simulink model "Estimador_DB_Caso_2"  (R2023a)
settings: Solver=VariableStepAuto  StartTime=0.0  StopTime=6  MaxStep=0.001  MinStep=0.0001  RelTol=1e-3  EnableMultiTasking=on
values from neighbouring files (symbols this model uses):
  A = [-1/(C1*R1) 1/(R1*C1);1/(C2*R1) -1/C2*(1/R1+1/R2)]    [MIMO_Real_Tanques.m]
  B = [1/C1 0;0 1/C2]    [MIMO_Real_Tanques.m]
  C = [1 0;0 1;0 1/R2]    [MIMO_Real_Tanques.m]
  D = [0 0;0 0;0 0]    [MIMO_Real_Tanques.m]
  K = place(A,B,PLC)    [MIMO_Real_Tanques.m]
  K0 = pinv(dcgain(ss(An,B,C,D)))*Y_inf*pinv(Q_inf)    [MIMO_Real_Tanques.m]
  Ke = place(A',C',PEE)'    [MIMO_Real_Tanques.m]
  Q1 = 3    [MIMO_Real_Tanques.m]
  Q2 = 1    [MIMO_Real_Tanques.m]
settings Model: Creator=54115  LastModifiedBy=franc
settings SolverCC: AlgebraicLoopSolver=TrustRegion
settings DataIOCC: ReturnWorkspaceOutputs=off
settings OptimizationCC: LifeSpan=inf
settings DebuggingCC: UnconnectedInputMsg=warning  UnconnectedOutputMsg=warning  UnconnectedLineMsg=warning  SFUnexpectedBacktrackingDiag=warning  SFNoUnconditionalDefaultTransitionDiag=warning  ArithmeticOperatorsInVariantConditions=warning
settings ModelReferenceCC: EnableRefExpFcnMdlSchedulingChecks=on
settings SFSimCC: SimUseLocalCustomCode=off  CustomCodeUndefinedFunction=UseInterfaceOnly
settings RTWCC: RTWUseLocalCustomCode=off
settings CodeAppCC: StateflowObjectComments=on
settings GRTTargetCC: TargetLangStandard=C89/C90 (ANSI)
settings ConfigComp: CovMetricSettings=dw  CovSaveCumulativeToWorkspaceVar=on  CovSaveSingleToWorkspaceVar=on  CovExternalEMLEnable=off

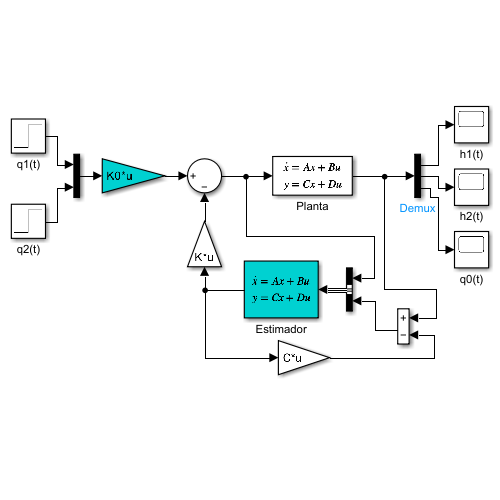
[thumbnail: Simulink's stored preview of the top-level diagram]
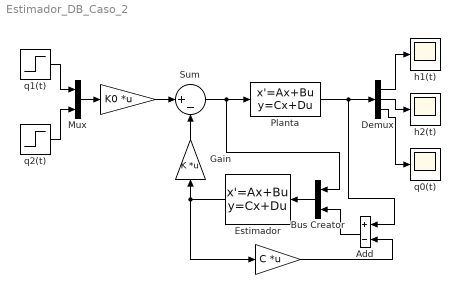
== system Estimador_DB_Caso_2 ==
  " " : Gain  Gain=K0  Multiplication=Matrix(K*u)
  "  " : Gain  Gain=C  Multiplication=Matrix(K*u)
  Add : Sum  Inputs=+-
  Bus Creator : BusCreator  Inputs=2
  Demux : Demux  Outputs=3
  Estimador : StateSpace  A=A  B=[B Ke]  C=eye(2)  D=[0 0 0 0 0;0 0 0 0 0]  InitialCondition=0
  Gain : Gain  Gain=K  Multiplication=Matrix(K*u)
  Mux : Mux  Inputs=2
  Planta : StateSpace  A=A  B=B  C=C  D=D  InitialCondition=0
  Sum : Sum  Inputs=|+-
  h1(t) : Scope
  h2(t) : Scope
  q0(t) : Scope
  q1(t) : Step  Time=0  After=Q1  SampleTime=0
  q2(t) : Step  Time=0  After=Q2  SampleTime=0
  wires:
  Estimador/1 -> Gain/1, "  "/1
  Bus Creator/1 -> Estimador/1
  Demux/1 -> h1(t)/1
  Mux/1 -> " "/1
  Demux/3 -> q0(t)/1
  q2(t)/1 -> Mux/2
  q1(t)/1 -> Mux/1
  Planta/1 -> Add/1, Demux/1
  Demux/2 -> h2(t)/1
  " "/1 -> Sum/1
  Gain/1 -> Sum/2
  "  "/1 -> Add/2
  Add/1 -> Bus Creator/2
  Sum/1 -> Bus Creator/1, Planta/1
